simulink model "engine_porebski"  (R2015a)
settings: Solver=ode45  StartTime=0.0  StopTime=100.0  RelTol=1e-3
values from neighbouring files (symbols this model uses):
  L = 0.1    [LP1.m]    (also in ParametryDoSymulacji.m; USImodel.m; wskaJak1.m; wskaJak2.m)
  R = 2    [LP1.m]    (also in ParametryDoSymulacji.m; USImodel.m; wskaJak1.m; wskaJak2.m)
undefined symbols (not defined in the file or in its folder): acc_bound, b, J, K, Ke, Kt, pos_bound, sigbuilder_block, u_max
settings Model: Creator=Kuba  LastModifiedBy=Student
settings DataIOCC: LimitDataPoints=off  SaveFormat=StructureWithTime
settings HardwareCC: ProdBitPerPointer=64  ProdLargestAtomicFloat=Float  ProdIntDivRoundTo=Zero  ProdEndianess=LittleEndian  ProdHWDeviceType=Specified
settings ModelReferenceCC: PropagateSignalLabelsOutOfModel=on
settings ConfigComp: CovMetricSettings=dw  CovHtmlReporting=on  CovSaveCumulativeToWorkspaceVar=on  CovSaveSingleToWorkspaceVar=on  CovExternalEMLEnable=off

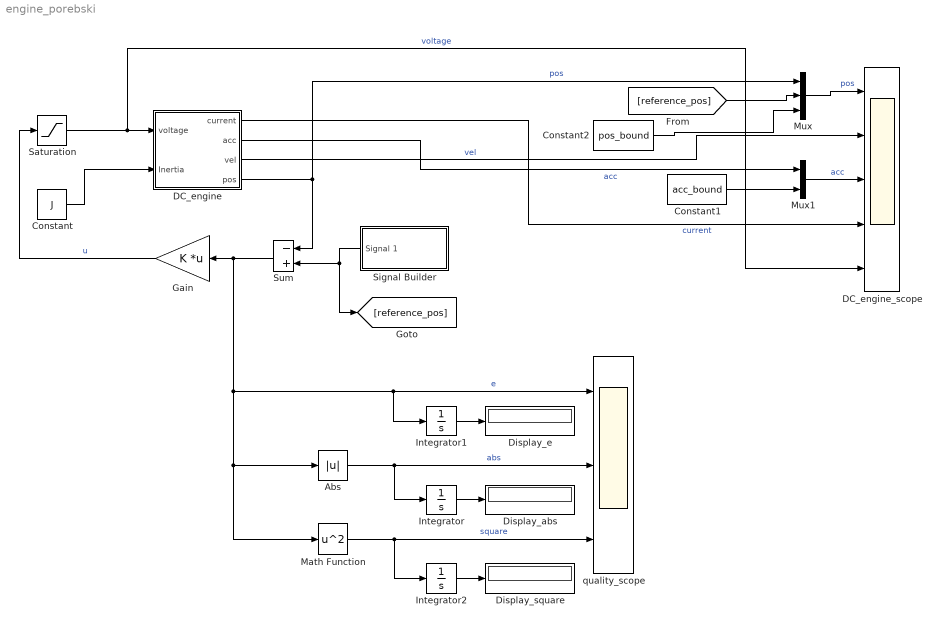
== system engine_porebski ==
  Abs : Abs
  Constant : Constant  Value=J
  Constant1 : Constant  Value=acc_bound
  Constant2 : Constant  Value=pos_bound
  DC_engine : Subsystem
  DC_engine_scope : Scope  NumInputPorts=5
      settings: YMin=-0.11208~-0.0518~-0.02594~-0.18812~-0.75267  YMax=0.41184~0.05163~0.06885~0.18755~0.7503  SaveName=Results
  Display_abs : Display
  Display_e : Display
  Display_square : Display
  Gain : Gain  Gain=K  Multiplication=Matrix(K*u)
  Integrator : Integrator
  Integrator1 : Integrator
  Integrator2 : Integrator
  Math Function : Math  Operator=square  SaturateOnIntegerOverflow=on
  Mux : Mux  Inputs=3
  Mux1 : Mux  Inputs=2
  Saturation : Saturate  UpperLimit=u_max  LowerLimit=-u_max
  Signal Builder : Subsystem  Tag=STV Subsys  LoadFcn=sigbuilder_block('load',[437.6 199.2 550.4 400 ]);  StartFcn=sigbuilder_block('start');  StopFcn=sigbuilder_block('stop');  ClipboardFcn=sigbuilder_block('clipboard');  mask(Sigbuilder block){}
      mask help: Simulink:masks:SigbuilderBlock_MD
      mask init:
      | if ~strcmp(get_param(bdroot(gcbh),'SimulationStatus'),'stopped') tuvar = sigbuilder_block('maskInit'); end
      settings: CopyFcn=sigbuilder_block('copy');  DeleteFcn=sigbuilder_block('delete');  ModelCloseFcn=sigbuilder_block('modelClose');  PreSaveFcn=sigbuilder_block('preSave');  PauseFcn=sigbuilder_block('pause');  ContinueFcn=sigbuilder_block('continue');  NameChangeFcn=sigbuilder_block('namechange');  OpenFcn=sigbuilder_block('open',[437.6 199.2 550.4 400 ]);  CloseFcn=sigbuilder_block('close');
      mask Display: plot(0, 0, 100, 100,[2, 2, 32, 32, 2], [68, 8, 8, 68, 68],[32, 2], [38, 38], [32, 19, 2],[53, 60, 44], [32, 17, 17, 2],[16, 16, 31, 31]);txt = getActiveGroup(gcbh);text(2, 100, txt,'verticalAlignment', 'top');
  Sum : Sum  Inputs=-+
  quality_scope : Scope  NumInputPorts=3
      settings: YMin=-0.37634~-0.03765~-0.01134  YMax=0.37515~0.33884~0.10205  SaveName=Results1
  wires:
  DC_engine/4(pos) -> Sum/1, Mux/1  "pos"
  DC_engine/3(vel) -> DC_engine_scope/2  "vel"
  DC_engine/1(current) -> DC_engine_scope/4  "current"
  Constant/1 -> DC_engine/2(Inertia)
  Saturation/1 -> DC_engine/1(voltage), DC_engine_scope/5  "voltage"
  Sum/1 -> Abs/1, Math Function/1, Integrator1/1, quality_scope/1, Gain/1  "e"
  Gain/1 -> Saturation/1  "u"
  Signal Builder/1(Signal 1) -> [reference_pos], Sum/2
  Mux/1 -> DC_engine_scope/1  "pos"
  [reference_pos] -> Mux/2
  Mux1/1 -> DC_engine_scope/3  "acc"
  DC_engine/2(acc) -> Mux1/1  "acc"
  Constant1/1 -> Mux1/2
  Constant2/1 -> Mux/3
  Integrator/1 -> Display_abs/1
  Abs/1 -> Integrator/1, quality_scope/2  "abs"
  Integrator1/1 -> Display_e/1
  Math Function/1 -> Integrator2/1, quality_scope/3  "square"
  Integrator2/1 -> Display_square/1

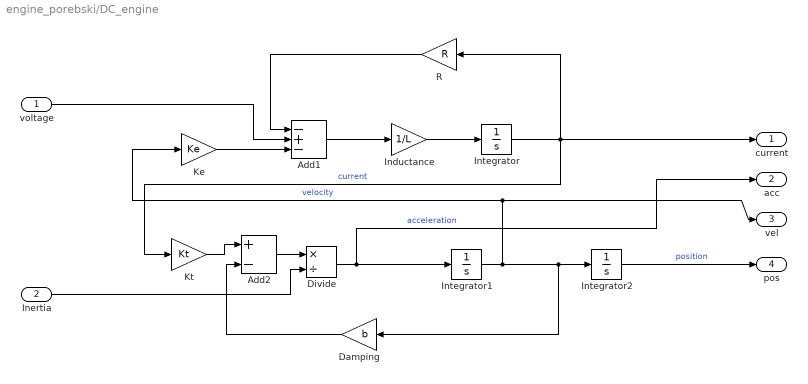
== system engine_porebski/DC_engine ==
  voltage : Inport
  Inertia : Inport  Port=2
  Add1 : Sum  Inputs=-+-
  Add2 : Sum  Inputs=+-
  Damping : Gain  Gain=b
  Divide : Product  Inputs=*/
  Inductance : Gain  Gain=1/L
  Integrator : Integrator
  Integrator1 : Integrator
  Integrator2 : Integrator
  Ke : Gain  Gain=Ke
  Kt : Gain  Gain=Kt
  R : Gain  Gain=R
  current : Outport
  acc : Outport  Port=2
  vel : Outport  Port=3
  pos : Outport  Port=4
  wires:
  voltage/1 -> Add1/2
  Integrator1/1 -> vel/1, Ke/1, Integrator2/1, Damping/1  "velocity"
  Damping/1 -> Add2/2
  Inductance/1 -> Integrator/1
  Divide/1 -> acc/1, Integrator1/1  "acceleration"
  Add2/1 -> Divide/1
  Kt/1 -> Add2/1
  Add1/1 -> Inductance/1
  Ke/1 -> Add1/3
  Integrator2/1 -> pos/1  "position"
  R/1 -> Add1/1
  Integrator/1 -> current/1, Kt/1, R/1  "current"
  Inertia/1 -> Divide/2

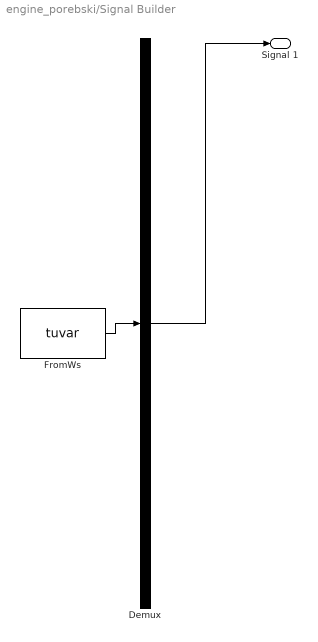
== system engine_porebski/Signal Builder ==
  Demux : Demux  Tag=STV Demux  Outputs=1
  FromWs : FromWorkspace  Tag=STV FromWs  VariableName=tuvar  SampleTime=0
      SigBuilderData=|
      | common.afterFinalStr = 'Extrapolate'
      | common.sampleTime = 0
      | dataSet.timeRange = [0 100]
      | dataSet.name = 'Group 1'
      | sbobj.Groups.Name = 'Group 1'
      | sbobj.Groups.Signals.Name = 'Signal 1'
      | sbobj.Groups.Signals.XData = [0 1 1 50 50 100]
      | sbobj.Groups.Signals.YData = [0 0 0.3 0.3 0 0]
      | sbobj.Groups.TimeRange = [0 100]
  Signal 1 : Outport  Tag=STV Outport
  wires:
  Demux/1 -> Signal 1/1
  FromWs/1 -> Demux/1
